simulink model "Servo_Validation"  (R2021a)
settings: Solver=VariableStepAuto  StartTime=0.0  StopTime=10  RelTol=1e-3
undefined symbols (not defined in the file): A_eta, A_x, B_u, C, F1, F2, F_eta, F_gamma, F_u, F_x, H_eta, H_gamma, H_u, H_x, params, y_d, z_0
settings Model: Creator=user  LastModifiedBy=sarmiento
settings SolverCC: AlgebraicLoopSolver=TrustRegion
settings DebuggingCC: SFMachineParentedDataDiag=warning

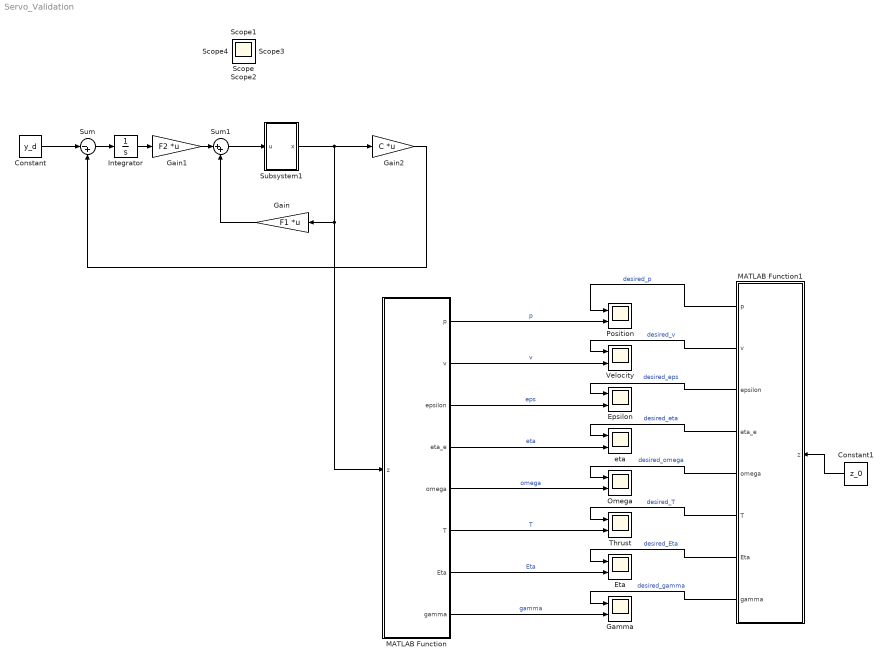
== system Servo_Validation ==
  Constant : Constant  Value=y_d
  Constant1 : Constant  Value=z_0
  Epsilon : Scope  NumInputPorts=2
  Eta : Scope  NumInputPorts=2
  Gain : Gain  Gain=F1  Multiplication=Matrix(K*u) (u vector)
  Gain1 : Gain  Gain=F2  Multiplication=Matrix(K*u) (u vector)
  Gain2 : Gain  Gain=C  Multiplication=Matrix(K*u) (u vector)
  Gamma : Scope  NumInputPorts=2
  Integrator : Integrator
  MATLAB Function : MATLAB Function  TreatAsAtomicUnit=on
  MATLAB Function1 : MATLAB Function  TreatAsAtomicUnit=on
  Omega : Scope  NumInputPorts=2
  Position : Scope  NumInputPorts=2
  Subsystem1 : Subsystem
  Sum : Sum  Inputs=|-+
  Sum1 : Sum  Inputs=|++
  Thrust : Scope  NumInputPorts=2
  Velocity : Scope  NumInputPorts=2
  eta : Scope  NumInputPorts=2
  Scope{,1..4} (5 alike) : Scope
  wires:
  Subsystem1/1(x) -> MATLAB Function/1(z), Gain/1, Gain2/1
  Sum1/1 -> Subsystem1/1(u)
  Gain/1 -> Sum1/2
  Gain2/1 -> Sum/2
  Constant/1 -> Sum/1
  Gain1/1 -> Sum1/1
  Sum/1 -> Integrator/1
  Integrator/1 -> Gain1/1
  MATLAB Function/6(T) -> Thrust/2  "T"
  MATLAB Function/1(p) -> Position/2  "p"
  MATLAB Function/5(omega) -> Omega/2  "omega"
  MATLAB Function/3(epsilon) -> Epsilon/2  "eps"
  MATLAB Function/7(Eta) -> Eta/2  "Eta"
  MATLAB Function/4(eta_e) -> eta/2  "eta"
  MATLAB Function/8(gamma) -> Gamma/2  "gamma"
  MATLAB Function/2(v) -> Velocity/2  "v"
  Constant1/1 -> MATLAB Function1/1(z)
  MATLAB Function1/1(p) -> Position/1  "desired_p"
  MATLAB Function1/2(v) -> Velocity/1  "desired_v"
  MATLAB Function1/3(epsilon) -> Epsilon/1  "desired_eps"
  MATLAB Function1/4(eta_e) -> eta/1  "desired_eta"
  MATLAB Function1/5(omega) -> Omega/1  "desired_omega"
  MATLAB Function1/6(T) -> Thrust/1  "desired_T"
  MATLAB Function1/7(Eta) -> Eta/1  "desired_Eta"
  MATLAB Function1/8(gamma) -> Gamma/1  "desired_gamma"

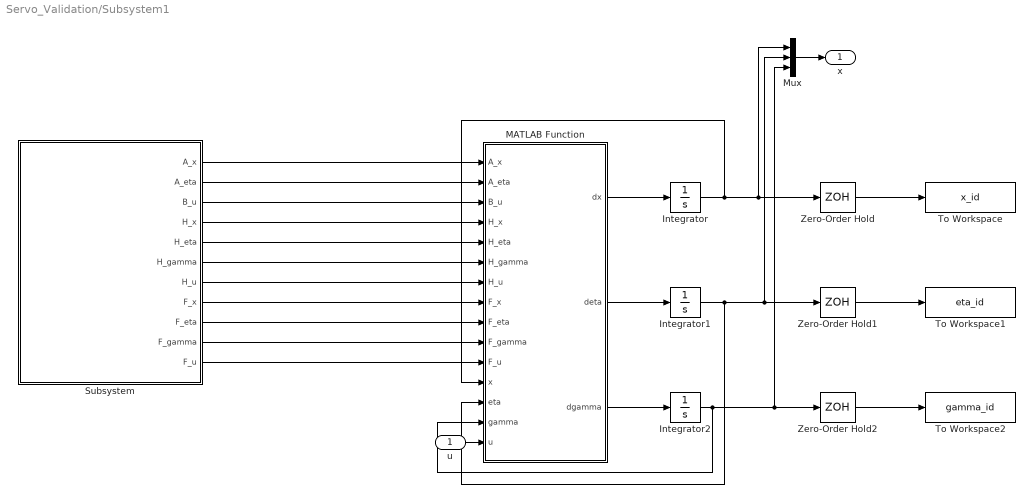
== system Servo_Validation/Subsystem1 ==
  u : Inport
  Integrator : Integrator  InitialCondition=params.x_0Taylor
  Integrator1 : Integrator  InitialCondition=params.eta_0
  Integrator2 : Integrator  InitialCondition=params.gamma_0
  MATLAB Function : MATLAB Function  TreatAsAtomicUnit=on
  Mux : Mux  Inputs=3
  Subsystem : Subsystem
  To Workspace : ToWorkspace  VariableName=x_id  SampleTime=-1
      settings: Save2DSignal=2-D array (concatenate along first dimension)
  To Workspace1 : ToWorkspace  VariableName=eta_id  SampleTime=-1
      settings: Save2DSignal=2-D array (concatenate along first dimension)
  To Workspace2 : ToWorkspace  VariableName=gamma_id  SampleTime=-1
      settings: Save2DSignal=2-D array (concatenate along first dimension)
  Zero-Order Hold : ZeroOrderHold  SampleTime=params.ST_id
  Zero-Order Hold1 : ZeroOrderHold  SampleTime=params.ST_id
  Zero-Order Hold2 : ZeroOrderHold  SampleTime=params.ST_id
  x : Outport
  wires:
  MATLAB Function/3(dgamma) -> Integrator2/1
  Subsystem/2(A_eta) -> MATLAB Function/2(A_eta)
  Integrator1/1 -> Mux/2, Zero-Order Hold1/1, MATLAB Function/13(eta)
  MATLAB Function/1(dx) -> Integrator/1
  u/1 -> MATLAB Function/15(u)
  Subsystem/8(F_x) -> MATLAB Function/8(F_x)
  Subsystem/3(B_u) -> MATLAB Function/3(B_u)
  Zero-Order Hold/1 -> To Workspace/1
  Subsystem/1(A_x) -> MATLAB Function/1(A_x)
  MATLAB Function/2(deta) -> Integrator1/1
  Subsystem/7(H_u) -> MATLAB Function/7(H_u)
  Zero-Order Hold2/1 -> To Workspace2/1
  Zero-Order Hold1/1 -> To Workspace1/1
  Subsystem/10(F_gamma) -> MATLAB Function/10(F_gamma)
  Subsystem/6(H_gamma) -> MATLAB Function/6(H_gamma)
  Subsystem/9(F_eta) -> MATLAB Function/9(F_eta)
  Subsystem/11(F_u) -> MATLAB Function/11(F_u)
  Subsystem/5(H_eta) -> MATLAB Function/5(H_eta)
  Integrator/1 -> MATLAB Function/12(x), Mux/1, Zero-Order Hold/1
  Subsystem/4(H_x) -> MATLAB Function/4(H_x)
  Integrator2/1 -> Zero-Order Hold2/1, Mux/3, MATLAB Function/14(gamma)
  Mux/1 -> x/1

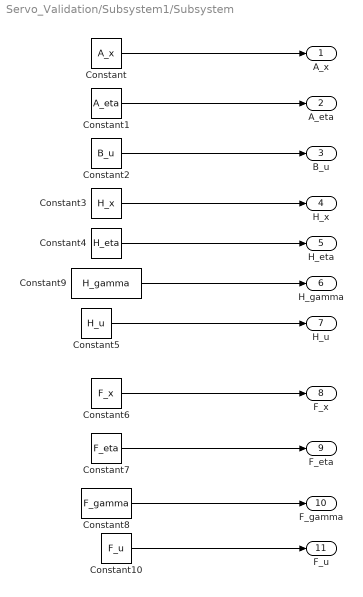
== system Servo_Validation/Subsystem1/Subsystem ==
  Constant : Constant  Value=A_x
  Constant1 : Constant  Value=A_eta
  Constant10 : Constant  Value=F_u
  Constant2 : Constant  Value=B_u
  Constant3 : Constant  Value=H_x
  Constant4 : Constant  Value=H_eta
  Constant5 : Constant  Value=H_u
  Constant6 : Constant  Value=F_x
  Constant7 : Constant  Value=F_eta
  Constant8 : Constant  Value=F_gamma
  Constant9 : Constant  Value=H_gamma
  A_x : Outport
  A_eta : Outport  Port=2
  B_u : Outport  Port=3
  H_x : Outport  Port=4
  H_eta : Outport  Port=5
  H_gamma : Outport  Port=6
  H_u : Outport  Port=7
  F_x : Outport  Port=8
  F_eta : Outport  Port=9
  F_gamma : Outport  Port=10
  F_u : Outport  Port=11
  wires:
  Constant2/1 -> B_u/1
  Constant6/1 -> F_x/1
  Constant3/1 -> H_x/1
  Constant/1 -> A_x/1
  Constant4/1 -> H_eta/1
  Constant5/1 -> H_u/1
  Constant7/1 -> F_eta/1
  Constant8/1 -> F_gamma/1
  Constant10/1 -> F_u/1
  Constant1/1 -> A_eta/1
  Constant9/1 -> H_gamma/1

== matlab function Servo_Validation/MATLAB Function1 ==
  data: z input; p output; v output; epsilon output; eta_e output; omega output; T output; Eta output; gamma output
function [p, v, epsilon, eta_e, omega, T, Eta, gamma] = fcn(z)
p = z(1:3);
v = z(4:6);
epsilon = z(7:9);
eta_e = z(10);
omega = z(11:13);
T = z(14);
Eta = z(15:32);
gamma = z(33:38);

== matlab function Servo_Validation/Subsystem1/MATLAB Function ==
  data: A_x input; A_eta input; B_u input; H_x input; H_eta input; H_gamma input; H_u input; F_x input; F_eta input; F_gamma input; F_u input; x input; eta input; gamma input; u input; dx output; deta output; dgamma output
function [dx,deta,dgamma] = fcn(A_x,A_eta,B_u,H_x,H_eta,H_gamma,H_u,F_x,F_eta,F_gamma,F_u,x,eta,gamma,u)

A_gamma = zeros(14,size(gamma, 1));

dx = A_x*x + A_eta*eta + A_gamma*gamma + B_u*u;

deta = H_x*x + H_eta*eta + H_gamma*gamma + H_u*u;

dgamma = F_x*x + F_eta*eta + F_gamma*gamma + F_u*u;
% epsilon = x (7:9,:);
% eta_e = sqrt(1-epsilon'*epsilon);
end

== matlab function Servo_Validation/MATLAB Function ==
  data: z input; p output; v output; epsilon output; eta_e output; omega output; T output; Eta output; gamma output
function [p, v, epsilon, eta_e, omega, T, Eta, gamma] = fcn(z)
p = z(1:3);
v = z(4:6);
epsilon = z(7:9);
eta_e = z(10);
omega = z(11:13);
T = z(14);
Eta = z(15:32);
gamma = z(33:38);
